simulink library "inp"  (R2021b)
settings: Solver=VariableStepAuto  StartTime=0.0  StopTime=10.0  RelTol=1e-3
undefined symbols (not defined in the file): C_TASK_5MS_S, FALSE, KINP_AcoreReadyToSlp_flg_ovrdflg, KINP_AcoreReadyToSlp_flg_ovrdval, KINP_AllowMovThd_OTA_enum_ovrdflg, KINP_AllowMovThd_OTA_enum_ovrdval, KINP_APSAngleTarget_Deg_ovrdflg, KINP_APSAngleTarget_Deg_ovrdval, KINP_APSDecReq_mps2_ovrdflg, KINP_APSDecReq_mps2_ovrdval, KINP_APSDecReqA_flg_ovrdflg, KINP_APSDecReqA_flg_ovrdval, KINP_APSDFLL_cm_ovrdflg, KINP_APSDFLL_cm_ovrdval, KINP_APSDFLR_cm_ovrdflg, KINP_APSDFLR_cm_ovrdval, KINP_APSDRLL_cm_ovrdflg, KINP_APSDRLL_cm_ovrdval, KINP_APSDRLR_cm_ovrdflg, KINP_APSDRLR_cm_ovrdval, KINP_APSExitCondition_enum_ovrdflg, KINP_APSExitCondition_enum_ovrdval, KINP_APSHWVer_enum_ovrdflg, KINP_APSHWVer_enum_ovrdval, KINP_APSProgressPCT_pct_ovrdflg, KINP_APSProgressPCT_pct_ovrdval, KINP_APSPwrReq_enum_ovrdflg, KINP_APSPwrReq_enum_ovrdval, KINP_APSReq_enum_ovrdflg, KINP_APSReq_enum_ovrdval, KINP_APSRQDisplay_enum_ovrdflg, KINP_APSRQDisplay_enum_ovrdval, KINP_APSRqEPASCtrl_flg_ovrdflg, KINP_APSRqEPASCtrl_flg_ovrdval, KINP_APSShiftPosnReq_enum_ovrdval, KINP_APSShiftPosnReq_enum_ovrflg, KINP_APSSpeedCMD_kph_ovrdval, KINP_APSSpeedCMD_kph_ovrflg, KINP_APSStaSystem_enum_ovrdflg, KINP_APSStaSystem_enum_ovrdval, KINP_APSSWVer_enum_ovrdflg, KINP_APSSWVer_enum_ovrdval, KINP_APSVMCReqA_flg_ovrdval, KINP_APSVMCReqA_flg_ovrflg, KINP_APSVRqEPASCtrl_flg_ovrdflg, KINP_APSVRqEPASCtrl_flg_ovrdval, KINP_AuxBattVolmV_mV_ovrdflg, KINP_AuxBattVolmV_mV_ovrdval, KINP_CAASSta_enum_ovrdflg, KINP_CAASSta_enum_ovrdval, KINP_CAASVMCReqA_flg_ovrdval, KINP_CAASVMCReqA_flg_ovrflg, KINP_CAN1BusOff_flg_ovrdflg, KINP_CAN1BusOff_flg_ovrdval, KINP_CAN2BusOff_flg_ovrdflg, KINP_CAN2BusOff_flg_ovrdval, KINP_CAN3BusOff_flg_ovrdflg, KINP_CAN3BusOff_flg_ovrdval, KINP_CAN4BusOff_flg_ovrdflg, KINP_CAN4BusOff_flg_ovrdval ... (+152)
libraries: FVT_lib x1037, hcu_lib x1
(part 15 of 34)

== system inp/INP/CAN1/SignalCheck/ESC5 ==
  BHAL_outputs : Inport
  inp_CanValid_bus : Inport  Port=2
  ACCAvail : FVT_lib/inp/can_signal_template  SystemSampleTime=-1  VariantActivationTime=update diagram  Latency=0  AutoFrameSizeCalculation=off
      link override defval: Value=KINP_ACCAvail_flg_defval
      link override ovrdflg: Value=KINP_ACCAvail_flg_ovrdflg
      link override ovrdval: Value=KINP_ACCAvail_flg_ovrdval
  AEBAvail : FVT_lib/inp/can_signal_template  SystemSampleTime=-1  VariantActivationTime=update diagram  Latency=0  AutoFrameSizeCalculation=off
      link override defval: Value=KINP_AEBAvail_flg_defval
      link override ovrdflg: Value=KINP_AEBAvail_flg_ovrdflg
      link override ovrdval: Value=KINP_AEBAvail_flg_ovrdval
  ActBrkLampSta : FVT_lib/inp/can_signal_template  SystemSampleTime=-1  VariantActivationTime=update diagram  Latency=0  AutoFrameSizeCalculation=off
      link override defval: Value=KINP_ActBrkLampSta_flg_defval
      link override ovrdflg: Value=KINP_ActBrkLampSta_flg_ovrdflg
      link override ovrdval: Value=KINP_ActBrkLampSta_flg_ovrdval
  BrkDiscTempSta : FVT_lib/inp/can_signal_template  SystemSampleTime=-1  VariantActivationTime=update diagram  Latency=0  AutoFrameSizeCalculation=off
      link override defval: Value=KINP_BrkDiscTempSta_flg_defval
      link override ovrdflg: Value=KINP_BrkDiscTempSta_flg_ovrdflg
      link override ovrdval: Value=KINP_BrkDiscTempSta_flg_ovrdval
  BrkPedalPos : FVT_lib/inp/can_signal_template  SystemSampleTime=-1  VariantActivationTime=update diagram  Latency=0  AutoFrameSizeCalculation=off
      link override defval: Value=KINP_BrkPedalPos_pct_defval
      link override ovrdflg: Value=KINP_BrkPedalPos_pct_ovrdflg
      link override ovrdval: Value=KINP_BrkPedalPos_pct_ovrdval
  BrkPedalPosSta : FVT_lib/inp/can_signal_template  SystemSampleTime=-1  VariantActivationTime=update diagram  Latency=0  AutoFrameSizeCalculation=off
      link override defval: Value=KINP_BrkPedalPosSta_flg_defval
      link override ovrdflg: Value=KINP_BrkPedalPosSta_flg_ovrdflg
      link override ovrdval: Value=KINP_BrkPedalPosSta_flg_ovrdval
  BrkSwSta : FVT_lib/inp/can_signal_template  SystemSampleTime=-1  VariantActivationTime=update diagram  Latency=0  AutoFrameSizeCalculation=off
      link override defval: Value=KINP_BrkSwSta_flg_defval
      link override ovrdflg: Value=KINP_BrkSwSta_flg_ovrdflg
      link override ovrdval: Value=KINP_BrkSwSta_flg_ovrdval
  BrkSwV : FVT_lib/inp/can_signal_template  SystemSampleTime=-1  VariantActivationTime=update diagram  Latency=0  AutoFrameSizeCalculation=off
      link override defval: Value=KINP_BrkSwV_flg_defval
      link override ovrdflg: Value=KINP_BrkSwV_flg_ovrdflg
      link override ovrdval: Value=KINP_BrkSwV_flg_ovrdval
  ESC5CS : FVT_lib/inp/can_signal_template  SystemSampleTime=-1  VariantActivationTime=update diagram  Latency=0  AutoFrameSizeCalculation=off
      link override defval: Value=KINP_ESC5CS_enum_defval
      link override ovrdflg: Value=KINP_ESC5CS_enum_ovrdflg
      link override ovrdval: Value=KINP_ESC5CS_enum_ovrdval
  ESC5CSErr : FVT_lib/inp/can_signal_template  SystemSampleTime=-1  VariantActivationTime=update diagram  Latency=0  AutoFrameSizeCalculation=off
      link override defval: Value=KINP_ESC5CSErr_flg_defval
      link override ovrdflg: Value=KINP_ESC5CSErr_flg_ovrdflg
      link override ovrdval: Value=KINP_ESC5CSErr_flg_ovrdval
  ESC5RC : FVT_lib/inp/can_signal_template  SystemSampleTime=-1  VariantActivationTime=update diagram  Latency=0  AutoFrameSizeCalculation=off
      link override defval: Value=KINP_ESC5RC_enum_defval
      link override ovrdflg: Value=KINP_ESC5RC_enum_ovrdflg
      link override ovrdval: Value=KINP_ESC5RC_enum_ovrdval
  ESC5RCErr : FVT_lib/inp/can_signal_template  SystemSampleTime=-1  VariantActivationTime=update diagram  Latency=0  AutoFrameSizeCalculation=off
      link override defval: Value=KINP_ESC5RCErr_flg_defval
      link override ovrdflg: Value=KINP_ESC5RCErr_flg_ovrdflg
      link override ovrdval: Value=KINP_ESC5RCErr_flg_ovrdval
  ESCADASSta : FVT_lib/inp/can_signal_template  SystemSampleTime=-1  VariantActivationTime=update diagram  Latency=0  AutoFrameSizeCalculation=off
      link override defval: Value=KINP_ESCADASSta_enum_defval
      link override ovrdflg: Value=KINP_ESCADASSta_enum_ovrdflg
      link override ovrdval: Value=KINP_ESCADASSta_enum_ovrdval
  ESCAPSSta : FVT_lib/inp/can_signal_template  SystemSampleTime=-1  VariantActivationTime=update diagram  Latency=0  AutoFrameSizeCalculation=off
      link override defval: Value=KINP_ESCAPSSta_enum_defval
      link override ovrdflg: Value=KINP_ESCAPSSta_enum_ovrdflg
      link override ovrdval: Value=KINP_ESCAPSSta_enum_ovrdval
  ESCStandstill : FVT_lib/inp/can_signal_template  SystemSampleTime=-1  VariantActivationTime=update diagram  Latency=0  AutoFrameSizeCalculation=off
      link override defval: Value=KINP_ESCStandstill_flg_defval
      link override ovrdflg: Value=KINP_ESCStandstill_flg_ovrdflg
      link override ovrdval: Value=KINP_ESCStandstill_flg_ovrdval
  FrRBCActive : FVT_lib/inp/can_signal_template  SystemSampleTime=-1  VariantActivationTime=update diagram  Latency=0  AutoFrameSizeCalculation=off
      link override defval: Value=KINP_FrRBCActive_flg_defval
      link override ovrdflg: Value=KINP_FrRBCActive_flg_ovrdflg
      link override ovrdval: Value=KINP_FrRBCActive_flg_ovrdval
  FrntAxlTrqReqBrk : FVT_lib/inp/can_signal_template  SystemSampleTime=-1  VariantActivationTime=update diagram  Latency=0  AutoFrameSizeCalculation=off
      link override defval: Value=KINP_FrntAxlTrqReqBrk_Nm_defval
      link override ovrdflg: Value=KINP_FrntAxlTrqReqBrk_Nm_ovrdflg
      link override ovrdval: Value=KINP_FrntAxlTrqReqBrk_Nm_ovrdval
  LatAccel : FVT_lib/inp/can_signal_template  SystemSampleTime=-1  VariantActivationTime=update diagram  Latency=0  AutoFrameSizeCalculation=off
      link override defval: Value=KINP_LatAccel_Gps_defval
      link override ovrdflg: Value=KINP_LatAccel_Gps_ovrdflg
      link override ovrdval: Value=KINP_LatAccel_Gps_ovrdval
  LatAccelV : FVT_lib/inp/can_signal_template  SystemSampleTime=-1  VariantActivationTime=update diagram  Latency=0  AutoFrameSizeCalculation=off
      link override defval: Value=KINP_LatAccelV_flg_defval
      link override ovrdflg: Value=KINP_LatAccelV_flg_ovrdflg
      link override ovrdval: Value=KINP_LatAccelV_flg_ovrdval
  LongAccel : FVT_lib/inp/can_signal_template  SystemSampleTime=-1  VariantActivationTime=update diagram  Latency=0  AutoFrameSizeCalculation=off
      link override defval: Value=KINP_LongAccel_Gps_defval
      link override ovrdflg: Value=KINP_LongAccel_Gps_ovrdflg
      link override ovrdval: Value=KINP_LongAccel_Gps_ovrdval
  LongAccelV : FVT_lib/inp/can_signal_template  SystemSampleTime=-1  VariantActivationTime=update diagram  Latency=0  AutoFrameSizeCalculation=off
      link override defval: Value=KINP_LongAccelV_flg_defval
      link override ovrdflg: Value=KINP_LongAccelV_flg_ovrdflg
      link override ovrdval: Value=KINP_LongAccelV_flg_ovrdval
  MCPressure : FVT_lib/inp/can_signal_template  SystemSampleTime=-1  VariantActivationTime=update diagram  Latency=0  AutoFrameSizeCalculation=off
      link override defval: Value=KINP_MCPressure_bar_defval
      link override ovrdflg: Value=KINP_MCPressure_bar_ovrdflg
      link override ovrdval: Value=KINP_MCPressure_bar_ovrdval
  MCPressureV : FVT_lib/inp/can_signal_template  SystemSampleTime=-1  VariantActivationTime=update diagram  Latency=0  AutoFrameSizeCalculation=off
      link override defval: Value=KINP_MCPressureV_flg_defval
      link override ovrdflg: Value=KINP_MCPressureV_flg_ovrdflg
      link override ovrdval: Value=KINP_MCPressureV_flg_ovrdval
  MeterIndVehSpeed : FVT_lib/inp/can_signal_template  SystemSampleTime=-1  VariantActivationTime=update diagram  Latency=0  AutoFrameSizeCalculation=off
      link override defval: Value=KINP_MeterIndVehSpeed_kph_defval
      link override ovrdflg: Value=KINP_MeterIndVehSpeed_kph_ovrdflg
      link override ovrdval: Value=KINP_MeterIndVehSpeed_kph_ovrdval
  RDCActive : FVT_lib/inp/can_signal_template  SystemSampleTime=-1  VariantActivationTime=update diagram  Latency=0  AutoFrameSizeCalculation=off
      link override defval: Value=KINP_RDCActive_enum_defval
      link override ovrdflg: Value=KINP_RDCActive_enum_ovrdflg
      link override ovrdval: Value=KINP_RDCActive_enum_ovrdval
  RearAxlTrqReqBrk : FVT_lib/inp/can_signal_template  SystemSampleTime=-1  VariantActivationTime=update diagram  Latency=0  AutoFrameSizeCalculation=off
      link override defval: Value=KINP_RearAxlTrqReqBrk_Nm_defval
      link override ovrdflg: Value=KINP_RearAxlTrqReqBrk_Nm_ovrdflg
      link override ovrdval: Value=KINP_RearAxlTrqReqBrk_Nm_ovrdval
  RrRBCActive : FVT_lib/inp/can_signal_template  SystemSampleTime=-1  VariantActivationTime=update diagram  Latency=0  AutoFrameSizeCalculation=off
      link override defval: Value=KINP_RrRBCActive_flg_defval
      link override ovrdflg: Value=KINP_RrRBCActive_flg_ovrdflg
      link override ovrdval: Value=KINP_RrRBCActive_flg_ovrdval
  Terminator_{1..29} (29 alike) : Terminator
  True_VHAL_ACCAvail_flg : Constant  Value=TRUE  OutDataTypeStr=boolean
  True_VHAL_AEBAvail_flg : Constant  Value=TRUE  OutDataTypeStr=boolean
  True_VHAL_ActBrkLampSta_flg : Constant  Value=TRUE  OutDataTypeStr=boolean
  True_VHAL_BrkDiscTempSta_flg : Constant  Value=TRUE  OutDataTypeStr=boolean
  True_VHAL_BrkPedalPosSta_flg : Constant  Value=TRUE  OutDataTypeStr=boolean
  True_VHAL_BrkPedalPos_pct : Constant  Value=TRUE  OutDataTypeStr=boolean
  True_VHAL_BrkSwSta_flg : Constant  Value=TRUE  OutDataTypeStr=boolean
  True_VHAL_BrkSwV_flg : Constant  Value=TRUE  OutDataTypeStr=boolean
  True_VHAL_ESC5CSErr_flg : Constant  Value=TRUE  OutDataTypeStr=boolean
  True_VHAL_ESC5CS_enum : Constant  Value=TRUE  OutDataTypeStr=boolean
  True_VHAL_ESC5RCErr_flg : Constant  Value=TRUE  OutDataTypeStr=boolean
  True_VHAL_ESC5RC_enum : Constant  Value=TRUE  OutDataTypeStr=boolean
  True_VHAL_ESCADASSta_enum : Constant  Value=TRUE  OutDataTypeStr=boolean
  True_VHAL_ESCAPSSta_enum : Constant  Value=TRUE  OutDataTypeStr=boolean
  True_VHAL_ESCStandstill_flg : Constant  Value=TRUE  OutDataTypeStr=boolean
  True_VHAL_FrRBCActive_flg : Constant  Value=TRUE  OutDataTypeStr=boolean
  True_VHAL_FrntAxlTrqReqBrk_Nm : Constant  Value=TRUE  OutDataTypeStr=boolean
  True_VHAL_LatAccelV_flg : Constant  Value=TRUE  OutDataTypeStr=boolean
  True_VHAL_LatAccel_Gps : Constant  Value=TRUE  OutDataTypeStr=boolean
  True_VHAL_LongAccelV_flg : Constant  Value=TRUE  OutDataTypeStr=boolean
  True_VHAL_LongAccel_Gps : Constant  Value=TRUE  OutDataTypeStr=boolean
  True_VHAL_MCPressureV_flg : Constant  Value=TRUE  OutDataTypeStr=boolean
  True_VHAL_MCPressure_bar : Constant  Value=TRUE  OutDataTypeStr=boolean
  True_VHAL_MeterIndVehSpeed_kph : Constant  Value=TRUE  OutDataTypeStr=boolean
  True_VHAL_RDCActive_enum : Constant  Value=TRUE  OutDataTypeStr=boolean
  True_VHAL_RearAxlTrqReqBrk_Nm : Constant  Value=TRUE  OutDataTypeStr=boolean
  True_VHAL_RrRBCActive_flg : Constant  Value=TRUE  OutDataTypeStr=boolean
  True_VHAL_YawRateV_flg : Constant  Value=TRUE  OutDataTypeStr=boolean
  True_VHAL_YawRate_degps : Constant  Value=TRUE  OutDataTypeStr=boolean
  YawRate : FVT_lib/inp/can_signal_template  SystemSampleTime=-1  VariantActivationTime=update diagram  Latency=0  AutoFrameSizeCalculation=off
      link override defval: Value=KINP_YawRate_degps_defval
      link override ovrdflg: Value=KINP_YawRate_degps_ovrdflg
      link override ovrdval: Value=KINP_YawRate_degps_ovrdval
  YawRateV : FVT_lib/inp/can_signal_template  SystemSampleTime=-1  VariantActivationTime=update diagram  Latency=0  AutoFrameSizeCalculation=off
      link override defval: Value=KINP_YawRateV_flg_defval
      link override ovrdflg: Value=KINP_YawRateV_flg_ovrdflg
      link override ovrdval: Value=KINP_YawRateV_flg_ovrdval
  slr1_{1..29} (29 alike) : BusSelector  OutputSignals=VINP_CANMsgValidESC5_flg
  slr_VHAL_ACCAvail_flg : BusSelector  OutputSignals=VHAL_ACCAvail_flg
  slr_VHAL_AEBAvail_flg : BusSelector  OutputSignals=VHAL_AEBAvail_flg
  slr_VHAL_ActBrkLampSta_flg : BusSelector  OutputSignals=VHAL_ActBrkLampSta_flg
  slr_VHAL_BrkDiscTempSta_flg : BusSelector  OutputSignals=VHAL_BrkDiscTempSta_flg
  slr_VHAL_BrkPedalPosSta_flg : BusSelector  OutputSignals=VHAL_BrkPedalPosSta_flg
  slr_VHAL_BrkPedalPos_pct : BusSelector  OutputSignals=VHAL_BrkPedalPos_pct
  slr_VHAL_BrkSwSta_flg : BusSelector  OutputSignals=VHAL_BrkSwSta_flg
  slr_VHAL_BrkSwV_flg : BusSelector  OutputSignals=VHAL_BrkSwV_flg
  slr_VHAL_ESC5CSErr_flg : BusSelector  OutputSignals=VHAL_ESC5CSErr_flg
  slr_VHAL_ESC5CS_enum : BusSelector  OutputSignals=VHAL_ESC5CS_enum
  slr_VHAL_ESC5RCErr_flg : BusSelector  OutputSignals=VHAL_ESC5RCErr_flg
  slr_VHAL_ESC5RC_enum : BusSelector  OutputSignals=VHAL_ESC5RC_enum
  slr_VHAL_ESCADASSta_enum : BusSelector  OutputSignals=VHAL_ESCADASSta_enum
  slr_VHAL_ESCAPSSta_enum : BusSelector  OutputSignals=VHAL_ESCAPSSta_enum
  slr_VHAL_ESCStandstill_flg : BusSelector  OutputSignals=VHAL_ESCStandstill_flg
  slr_VHAL_FrRBCActive_flg : BusSelector  OutputSignals=VHAL_FrRBCActive_flg
  slr_VHAL_FrntAxlTrqReqBrk_Nm : BusSelector  OutputSignals=VHAL_FrntAxlTrqReqBrk_Nm
  slr_VHAL_LatAccelV_flg : BusSelector  OutputSignals=VHAL_LatAccelV_flg
  slr_VHAL_LatAccel_Gps : BusSelector  OutputSignals=VHAL_LatAccel_Gps
  slr_VHAL_LongAccelV_flg : BusSelector  OutputSignals=VHAL_LongAccelV_flg
  slr_VHAL_LongAccel_Gps : BusSelector  OutputSignals=VHAL_LongAccel_Gps
  slr_VHAL_MCPressureV_flg : BusSelector  OutputSignals=VHAL_MCPressureV_flg
  slr_VHAL_MCPressure_bar : BusSelector  OutputSignals=VHAL_MCPressure_bar
  slr_VHAL_MeterIndVehSpeed_kph : BusSelector  OutputSignals=VHAL_MeterIndVehSpeed_kph
  slr_VHAL_RDCActive_enum : BusSelector  OutputSignals=VHAL_RDCActive_enum
  slr_VHAL_RearAxlTrqReqBrk_Nm : BusSelector  OutputSignals=VHAL_RearAxlTrqReqBrk_Nm
  slr_VHAL_RrRBCActive_flg : BusSelector  OutputSignals=VHAL_RrRBCActive_flg
  slr_VHAL_YawRateV_flg : BusSelector  OutputSignals=VHAL_YawRateV_flg
  slr_VHAL_YawRate_degps : BusSelector  OutputSignals=VHAL_YawRate_degps
  VINP_ESC5CSErr_flg : Outport
  VINP_ESC5RCErr_flg : Outport  Port=2
  VINP_ACCAvail_flg : Outport  Port=3
  VINP_AEBAvail_flg : Outport  Port=4
  VINP_ActBrkLampSta_flg : Outport  Port=5
  VINP_BrkDiscTempSta_flg : Outport  Port=6
  VINP_BrkPedalPos_pct : Outport  Port=7
  VINP_BrkPedalPosSta_flg : Outport  Port=8
  VINP_BrkSwSta_flg : Outport  Port=9
  VINP_BrkSwV_flg : Outport  Port=10
  VINP_ESC5CS_enum : Outport  Port=11
  VINP_ESC5RC_enum : Outport  Port=12
  VINP_ESCADASSta_enum : Outport  Port=13
  VINP_ESCAPSSta_enum : Outport  Port=14
  VINP_ESCStandstill_flg : Outport  Port=15
  VINP_FrRBCActive_flg : Outport  Port=16
  VINP_FrntAxlTrqReqBrk_Nm : Outport  Port=17
  VINP_LatAccel_Gps : Outport  Port=18
  VINP_LatAccelV_flg : Outport  Port=19
  VINP_LongAccel_Gps : Outport  Port=20
  VINP_LongAccelV_flg : Outport  Port=21
  VINP_MCPressure_bar : Outport  Port=22
  VINP_MCPressureV_flg : Outport  Port=23
  VINP_MeterIndVehSpeed_kph : Outport  Port=24
  VINP_RDCActive_enum : Outport  Port=25
  VINP_RearAxlTrqReqBrk_Nm : Outport  Port=26
  VINP_RrRBCActive_flg : Outport  Port=27
  VINP_YawRate_degps : Outport  Port=28
  VINP_YawRateV_flg : Outport  Port=29
  wires:
  BHAL_outputs/1 -> [BHAL_outputs]
  inp_CanValid_bus/1 -> [inp_CanValid_bus]
  [BHAL_outputs] -> slr_VHAL_ESC5CSErr_flg/1
  slr_VHAL_ESC5CSErr_flg/1 -> ESC5CSErr/1  "<VHAL_ESC5CSErr_flg>"
  True_VHAL_ESC5CSErr_flg/1 -> ESC5CSErr/2
  [inp_CanValid_bus] -> slr1_1/1
  slr1_1/1 -> ESC5CSErr/3  "<VINP_CANMsgValidESC5_flg>"
  ESC5CSErr/1 -> VINP_ESC5CSErr_flg/1  "VINP_ESC5CSErr_flg"
  ESC5CSErr/2 -> Terminator_1/1
  [BHAL_outputs] -> slr_VHAL_ESC5RCErr_flg/1
  slr_VHAL_ESC5RCErr_flg/1 -> ESC5RCErr/1  "<VHAL_ESC5RCErr_flg>"
  True_VHAL_ESC5RCErr_flg/1 -> ESC5RCErr/2
  [inp_CanValid_bus] -> slr1_2/1
  slr1_2/1 -> ESC5RCErr/3  "<VINP_CANMsgValidESC5_flg>"
  ESC5RCErr/1 -> VINP_ESC5RCErr_flg/1  "VINP_ESC5RCErr_flg"
  ESC5RCErr/2 -> Terminator_2/1
  [BHAL_outputs] -> slr_VHAL_ACCAvail_flg/1
  slr_VHAL_ACCAvail_flg/1 -> ACCAvail/1  "<VHAL_ACCAvail_flg>"
  True_VHAL_ACCAvail_flg/1 -> ACCAvail/2
  [inp_CanValid_bus] -> slr1_3/1
  slr1_3/1 -> ACCAvail/3  "<VINP_CANMsgValidESC5_flg>"
  ACCAvail/1 -> VINP_ACCAvail_flg/1  "VINP_ACCAvail_flg"
  ACCAvail/2 -> Terminator_3/1
  [BHAL_outputs] -> slr_VHAL_AEBAvail_flg/1
  slr_VHAL_AEBAvail_flg/1 -> AEBAvail/1  "<VHAL_AEBAvail_flg>"
  True_VHAL_AEBAvail_flg/1 -> AEBAvail/2
  [inp_CanValid_bus] -> slr1_4/1
  slr1_4/1 -> AEBAvail/3  "<VINP_CANMsgValidESC5_flg>"
  AEBAvail/1 -> VINP_AEBAvail_flg/1  "VINP_AEBAvail_flg"
  AEBAvail/2 -> Terminator_4/1
  [BHAL_outputs] -> slr_VHAL_ActBrkLampSta_flg/1
  slr_VHAL_ActBrkLampSta_flg/1 -> ActBrkLampSta/1  "<VHAL_ActBrkLampSta_flg>"
  True_VHAL_ActBrkLampSta_flg/1 -> ActBrkLampSta/2
  [inp_CanValid_bus] -> slr1_5/1
  slr1_5/1 -> ActBrkLampSta/3  "<VINP_CANMsgValidESC5_flg>"
  ActBrkLampSta/1 -> VINP_ActBrkLampSta_flg/1  "VINP_ActBrkLampSta_flg"
  ActBrkLampSta/2 -> Terminator_5/1
  [BHAL_outputs] -> slr_VHAL_BrkDiscTempSta_flg/1
  slr_VHAL_BrkDiscTempSta_flg/1 -> BrkDiscTempSta/1  "<VHAL_BrkDiscTempSta_flg>"
  True_VHAL_BrkDiscTempSta_flg/1 -> BrkDiscTempSta/2
  [inp_CanValid_bus] -> slr1_6/1
  slr1_6/1 -> BrkDiscTempSta/3  "<VINP_CANMsgValidESC5_flg>"
  BrkDiscTempSta/1 -> VINP_BrkDiscTempSta_flg/1  "VINP_BrkDiscTempSta_flg"
  BrkDiscTempSta/2 -> Terminator_6/1
  [BHAL_outputs] -> slr_VHAL_BrkPedalPos_pct/1
  slr_VHAL_BrkPedalPos_pct/1 -> BrkPedalPos/1  "<VHAL_BrkPedalPos_pct>"
  True_VHAL_BrkPedalPos_pct/1 -> BrkPedalPos/2
  [inp_CanValid_bus] -> slr1_7/1
  slr1_7/1 -> BrkPedalPos/3  "<VINP_CANMsgValidESC5_flg>"
  BrkPedalPos/1 -> VINP_BrkPedalPos_pct/1  "VINP_BrkPedalPos_pct"
  BrkPedalPos/2 -> Terminator_7/1
  [BHAL_outputs] -> slr_VHAL_BrkPedalPosSta_flg/1
  slr_VHAL_BrkPedalPosSta_flg/1 -> BrkPedalPosSta/1  "<VHAL_BrkPedalPosSta_flg>"
  True_VHAL_BrkPedalPosSta_flg/1 -> BrkPedalPosSta/2
  [inp_CanValid_bus] -> slr1_8/1
  slr1_8/1 -> BrkPedalPosSta/3  "<VINP_CANMsgValidESC5_flg>"
  BrkPedalPosSta/1 -> VINP_BrkPedalPosSta_flg/1  "VINP_BrkPedalPosSta_flg"
  BrkPedalPosSta/2 -> Terminator_8/1
  [BHAL_outputs] -> slr_VHAL_BrkSwSta_flg/1
  slr_VHAL_BrkSwSta_flg/1 -> BrkSwSta/1  "<VHAL_BrkSwSta_flg>"
  True_VHAL_BrkSwSta_flg/1 -> BrkSwSta/2
  [inp_CanValid_bus] -> slr1_9/1
  slr1_9/1 -> BrkSwSta/3  "<VINP_CANMsgValidESC5_flg>"
  BrkSwSta/1 -> VINP_BrkSwSta_flg/1  "VINP_BrkSwSta_flg"
  BrkSwSta/2 -> Terminator_9/1
  [BHAL_outputs] -> slr_VHAL_BrkSwV_flg/1
  slr_VHAL_BrkSwV_flg/1 -> BrkSwV/1  "<VHAL_BrkSwV_flg>"
  True_VHAL_BrkSwV_flg/1 -> BrkSwV/2
  [inp_CanValid_bus] -> slr1_10/1
  slr1_10/1 -> BrkSwV/3  "<VINP_CANMsgValidESC5_flg>"
  BrkSwV/1 -> VINP_BrkSwV_flg/1  "VINP_BrkSwV_flg"
  BrkSwV/2 -> Terminator_10/1
  [BHAL_outputs] -> slr_VHAL_ESC5CS_enum/1
  slr_VHAL_ESC5CS_enum/1 -> ESC5CS/1  "<VHAL_ESC5CS_enum>"
  True_VHAL_ESC5CS_enum/1 -> ESC5CS/2
  [inp_CanValid_bus] -> slr1_11/1
  slr1_11/1 -> ESC5CS/3  "<VINP_CANMsgValidESC5_flg>"
  ESC5CS/1 -> VINP_ESC5CS_enum/1  "VINP_ESC5CS_enum"
  ESC5CS/2 -> Terminator_11/1
  [BHAL_outputs] -> slr_VHAL_ESC5RC_enum/1
  slr_VHAL_ESC5RC_enum/1 -> ESC5RC/1  "<VHAL_ESC5RC_enum>"
  True_VHAL_ESC5RC_enum/1 -> ESC5RC/2
  [inp_CanValid_bus] -> slr1_12/1
  slr1_12/1 -> ESC5RC/3  "<VINP_CANMsgValidESC5_flg>"
  ESC5RC/1 -> VINP_ESC5RC_enum/1  "VINP_ESC5RC_enum"
  ESC5RC/2 -> Terminator_12/1
  [BHAL_outputs] -> slr_VHAL_ESCADASSta_enum/1
  slr_VHAL_ESCADASSta_enum/1 -> ESCADASSta/1  "<VHAL_ESCADASSta_enum>"
  True_VHAL_ESCADASSta_enum/1 -> ESCADASSta/2
  [inp_CanValid_bus] -> slr1_13/1
  slr1_13/1 -> ESCADASSta/3  "<VINP_CANMsgValidESC5_flg>"
  ESCADASSta/1 -> VINP_ESCADASSta_enum/1  "VINP_ESCADASSta_enum"
  ESCADASSta/2 -> Terminator_13/1
  [BHAL_outputs] -> slr_VHAL_ESCAPSSta_enum/1
  slr_VHAL_ESCAPSSta_enum/1 -> ESCAPSSta/1  "<VHAL_ESCAPSSta_enum>"
  True_VHAL_ESCAPSSta_enum/1 -> ESCAPSSta/2
  [inp_CanValid_bus] -> slr1_14/1
  slr1_14/1 -> ESCAPSSta/3  "<VINP_CANMsgValidESC5_flg>"
  ESCAPSSta/1 -> VINP_ESCAPSSta_enum/1  "VINP_ESCAPSSta_enum"
  ESCAPSSta/2 -> Terminator_14/1
  [BHAL_outputs] -> slr_VHAL_ESCStandstill_flg/1
  slr_VHAL_ESCStandstill_flg/1 -> ESCStandstill/1  "<VHAL_ESCStandstill_flg>"
  True_VHAL_ESCStandstill_flg/1 -> ESCStandstill/2
  [inp_CanValid_bus] -> slr1_15/1
  slr1_15/1 -> ESCStandstill/3  "<VINP_CANMsgValidESC5_flg>"
  ESCStandstill/1 -> VINP_ESCStandstill_flg/1  "VINP_ESCStandstill_flg"
  ESCStandstill/2 -> Terminator_15/1
  [BHAL_outputs] -> slr_VHAL_FrRBCActive_flg/1
  slr_VHAL_FrRBCActive_flg/1 -> FrRBCActive/1  "<VHAL_FrRBCActive_flg>"
  True_VHAL_FrRBCActive_flg/1 -> FrRBCActive/2
  [inp_CanValid_bus] -> slr1_16/1
  slr1_16/1 -> FrRBCActive/3  "<VINP_CANMsgValidESC5_flg>"
  FrRBCActive/1 -> VINP_FrRBCActive_flg/1  "VINP_FrRBCActive_flg"
  FrRBCActive/2 -> Terminator_16/1
  [BHAL_outputs] -> slr_VHAL_FrntAxlTrqReqBrk_Nm/1
  slr_VHAL_FrntAxlTrqReqBrk_Nm/1 -> FrntAxlTrqReqBrk/1  "<VHAL_FrntAxlTrqReqBrk_Nm>"
  True_VHAL_FrntAxlTrqReqBrk_Nm/1 -> FrntAxlTrqReqBrk/2
  [inp_CanValid_bus] -> slr1_17/1
  slr1_17/1 -> FrntAxlTrqReqBrk/3  "<VINP_CANMsgValidESC5_flg>"
  FrntAxlTrqReqBrk/1 -> VINP_FrntAxlTrqReqBrk_Nm/1  "VINP_FrntAxlTrqReqBrk_Nm"
  FrntAxlTrqReqBrk/2 -> Terminator_17/1
  [BHAL_outputs] -> slr_VHAL_LatAccel_Gps/1
  slr_VHAL_LatAccel_Gps/1 -> LatAccel/1  "<VHAL_LatAccel_Gps>"
  True_VHAL_LatAccel_Gps/1 -> LatAccel/2
  [inp_CanValid_bus] -> slr1_18/1
  slr1_18/1 -> LatAccel/3  "<VINP_CANMsgValidESC5_flg>"
  LatAccel/1 -> VINP_LatAccel_Gps/1  "VINP_LatAccel_Gps"
  LatAccel/2 -> Terminator_18/1
  [BHAL_outputs] -> slr_VHAL_LatAccelV_flg/1
  slr_VHAL_LatAccelV_flg/1 -> LatAccelV/1  "<VHAL_LatAccelV_flg>"
  True_VHAL_LatAccelV_flg/1 -> LatAccelV/2
  [inp_CanValid_bus] -> slr1_19/1
  slr1_19/1 -> LatAccelV/3  "<VINP_CANMsgValidESC5_flg>"
  LatAccelV/1 -> VINP_LatAccelV_flg/1  "VINP_LatAccelV_flg"
  LatAccelV/2 -> Terminator_19/1
  [BHAL_outputs] -> slr_VHAL_LongAccel_Gps/1
  slr_VHAL_LongAccel_Gps/1 -> LongAccel/1  "<VHAL_LongAccel_Gps>"
  True_VHAL_LongAccel_Gps/1 -> LongAccel/2
  [inp_CanValid_bus] -> slr1_20/1
  slr1_20/1 -> LongAccel/3  "<VINP_CANMsgValidESC5_flg>"
  LongAccel/1 -> VINP_LongAccel_Gps/1  "VINP_LongAccel_Gps"
  LongAccel/2 -> Terminator_20/1
  [BHAL_outputs] -> slr_VHAL_LongAccelV_flg/1
  slr_VHAL_LongAccelV_flg/1 -> LongAccelV/1  "<VHAL_LongAccelV_flg>"
  True_VHAL_LongAccelV_flg/1 -> LongAccelV/2
  [inp_CanValid_bus] -> slr1_21/1
  slr1_21/1 -> LongAccelV/3  "<VINP_CANMsgValidESC5_flg>"
  LongAccelV/1 -> VINP_LongAccelV_flg/1  "VINP_LongAccelV_flg"
  LongAccelV/2 -> Terminator_21/1
  [BHAL_outputs] -> slr_VHAL_MCPressure_bar/1
  slr_VHAL_MCPressure_bar/1 -> MCPressure/1  "<VHAL_MCPressure_bar>"
  True_VHAL_MCPressure_bar/1 -> MCPressure/2
  [inp_CanValid_bus] -> slr1_22/1
  slr1_22/1 -> MCPressure/3  "<VINP_CANMsgValidESC5_flg>"
  MCPressure/1 -> VINP_MCPressure_bar/1  "VINP_MCPressure_bar"
  MCPressure/2 -> Terminator_22/1
  [BHAL_outputs] -> slr_VHAL_MCPressureV_flg/1
  slr_VHAL_MCPressureV_flg/1 -> MCPressureV/1  "<VHAL_MCPressureV_flg>"
  True_VHAL_MCPressureV_flg/1 -> MCPressureV/2
  [inp_CanValid_bus] -> slr1_23/1
  slr1_23/1 -> MCPressureV/3  "<VINP_CANMsgValidESC5_flg>"
  MCPressureV/1 -> VINP_MCPressureV_flg/1  "VINP_MCPressureV_flg"
  MCPressureV/2 -> Terminator_23/1
  [BHAL_outputs] -> slr_VHAL_MeterIndVehSpeed_kph/1
  slr_VHAL_MeterIndVehSpeed_kph/1 -> MeterIndVehSpeed/1  "<VHAL_MeterIndVehSpeed_kph>"
  True_VHAL_MeterIndVehSpeed_kph/1 -> MeterIndVehSpeed/2
  [inp_CanValid_bus] -> slr1_24/1
  slr1_24/1 -> MeterIndVehSpeed/3  "<VINP_CANMsgValidESC5_flg>"
  MeterIndVehSpeed/1 -> VINP_MeterIndVehSpeed_kph/1  "VINP_MeterIndVehSpeed_kph"
  MeterIndVehSpeed/2 -> Terminator_24/1
  [BHAL_outputs] -> slr_VHAL_RDCActive_enum/1
  slr_VHAL_RDCActive_enum/1 -> RDCActive/1  "<VHAL_RDCActive_enum>"
  True_VHAL_RDCActive_enum/1 -> RDCActive/2
  [inp_CanValid_bus] -> slr1_25/1
  slr1_25/1 -> RDCActive/3  "<VINP_CANMsgValidESC5_flg>"
  RDCActive/1 -> VINP_RDCActive_enum/1  "VINP_RDCActive_enum"
  RDCActive/2 -> Terminator_25/1
  [BHAL_outputs] -> slr_VHAL_RearAxlTrqReqBrk_Nm/1
  slr_VHAL_RearAxlTrqReqBrk_Nm/1 -> RearAxlTrqReqBrk/1  "<VHAL_RearAxlTrqReqBrk_Nm>"
  True_VHAL_RearAxlTrqReqBrk_Nm/1 -> RearAxlTrqReqBrk/2
  [inp_CanValid_bus] -> slr1_26/1
  slr1_26/1 -> RearAxlTrqReqBrk/3  "<VINP_CANMsgValidESC5_flg>"
  RearAxlTrqReqBrk/1 -> VINP_RearAxlTrqReqBrk_Nm/1  "VINP_RearAxlTrqReqBrk_Nm"
  RearAxlTrqReqBrk/2 -> Terminator_26/1
  [BHAL_outputs] -> slr_VHAL_RrRBCActive_flg/1
  slr_VHAL_RrRBCActive_flg/1 -> RrRBCActive/1  "<VHAL_RrRBCActive_flg>"
  True_VHAL_RrRBCActive_flg/1 -> RrRBCActive/2
  [inp_CanValid_bus] -> slr1_27/1
  slr1_27/1 -> RrRBCActive/3  "<VINP_CANMsgValidESC5_flg>"
  RrRBCActive/1 -> VINP_RrRBCActive_flg/1  "VINP_RrRBCActive_flg"
  RrRBCActive/2 -> Terminator_27/1
  [BHAL_outputs] -> slr_VHAL_YawRate_degps/1
  slr_VHAL_YawRate_degps/1 -> YawRate/1  "<VHAL_YawRate_degps>"
  True_VHAL_YawRate_degps/1 -> YawRate/2
  [inp_CanValid_bus] -> slr1_28/1
  slr1_28/1 -> YawRate/3  "<VINP_CANMsgValidESC5_flg>"
  YawRate/1 -> VINP_YawRate_degps/1  "VINP_YawRate_degps"
  YawRate/2 -> Terminator_28/1
  [BHAL_outputs] -> slr_VHAL_YawRateV_flg/1
  slr_VHAL_YawRateV_flg/1 -> YawRateV/1  "<VHAL_YawRateV_flg>"
  True_VHAL_YawRateV_flg/1 -> YawRateV/2
  [inp_CanValid_bus] -> slr1_29/1
  slr1_29/1 -> YawRateV/3  "<VINP_CANMsgValidESC5_flg>"
  YawRateV/1 -> VINP_YawRateV_flg/1  "VINP_YawRateV_flg"
  YawRateV/2 -> Terminator_29/1

== system inp/INP/CAN1/SignalCheck/eBST1 ==
  BHAL_outputs : Inport
  inp_CanValid_bus : Inport  Port=2
  LowBrakeFluidSta : FVT_lib/inp/can_signal_template  SystemSampleTime=-1  VariantActivationTime=update diagram  Latency=0  AutoFrameSizeCalculation=off
      link override defval: Value=KINP_LowBrakeFluidSta_flg_defval
      link override ovrdflg: Value=KINP_LowBrakeFluidSta_flg_ovrdflg
      link override ovrdval: Value=KINP_LowBrakeFluidSta_flg_ovrdval
  Terminator_{1..4} (4 alike) : Terminator
  True_VHAL_LowBrakeFluidSta_flg : Constant  Value=TRUE  OutDataTypeStr=boolean
  True_VHAL_eBSTAmberWnlmpSta_flg : Constant  Value=TRUE  OutDataTypeStr=boolean
  True_VHAL_eBSTBeepReq_flg : Constant  Value=TRUE  OutDataTypeStr=boolean
  True_VHAL_eBSTRedWnlmpSta_flg : Constant  Value=TRUE  OutDataTypeStr=boolean
  eBSTAmberWnlmpSta : FVT_lib/inp/can_signal_template  SystemSampleTime=-1  VariantActivationTime=update diagram  Latency=0  AutoFrameSizeCalculation=off
      link override defval: Value=KINP_eBSTAmberWnlmpSta_flg_defval
      link override ovrdflg: Value=KINP_eBSTAmberWnlmpSta_flg_ovrdflg
      link override ovrdval: Value=KINP_eBSTAmberWnlmpSta_flg_ovrdval
  eBSTBeepReq : FVT_lib/inp/can_signal_template  SystemSampleTime=-1  VariantActivationTime=update diagram  Latency=0  AutoFrameSizeCalculation=off
      link override defval: Value=KINP_eBSTBeepReq_flg_defval
      link override ovrdflg: Value=KINP_eBSTBeepReq_flg_ovrdflg
      link override ovrdval: Value=KINP_eBSTBeepReq_flg_ovrdval
  eBSTRedWnlmpSta : FVT_lib/inp/can_signal_template  SystemSampleTime=-1  VariantActivationTime=update diagram  Latency=0  AutoFrameSizeCalculation=off
      link override defval: Value=KINP_eBSTRedWnlmpSta_flg_defval
      link override ovrdflg: Value=KINP_eBSTRedWnlmpSta_flg_ovrdflg
      link override ovrdval: Value=KINP_eBSTRedWnlmpSta_flg_ovrdval
  slr1_{1..4} (4 alike) : BusSelector  OutputSignals=VINP_CANMsgValideBST1_flg
  slr_VHAL_LowBrakeFluidSta_flg : BusSelector  OutputSignals=VHAL_LowBrakeFluidSta_flg
  slr_VHAL_eBSTAmberWnlmpSta_flg : BusSelector  OutputSignals=VHAL_eBSTAmberWnlmpSta_flg
  slr_VHAL_eBSTBeepReq_flg : BusSelector  OutputSignals=VHAL_eBSTBeepReq_flg
  slr_VHAL_eBSTRedWnlmpSta_flg : BusSelector  OutputSignals=VHAL_eBSTRedWnlmpSta_flg
  VINP_LowBrakeFluidSta_flg : Outport
  VINP_eBSTAmberWnlmpSta_flg : Outport  Port=2
  VINP_eBSTBeepReq_flg : Outport  Port=3
  VINP_eBSTRedWnlmpSta_flg : Outport  Port=4
  wires:
  BHAL_outputs/1 -> [BHAL_outputs]
  inp_CanValid_bus/1 -> [inp_CanValid_bus]
  [BHAL_outputs] -> slr_VHAL_LowBrakeFluidSta_flg/1
  slr_VHAL_LowBrakeFluidSta_flg/1 -> LowBrakeFluidSta/1  "<VHAL_LowBrakeFluidSta_flg>"
  True_VHAL_LowBrakeFluidSta_flg/1 -> LowBrakeFluidSta/2
  [inp_CanValid_bus] -> slr1_1/1
  slr1_1/1 -> LowBrakeFluidSta/3  "<VINP_CANMsgValideBST1_flg>"
  LowBrakeFluidSta/1 -> VINP_LowBrakeFluidSta_flg/1  "VINP_LowBrakeFluidSta_flg"
  LowBrakeFluidSta/2 -> Terminator_1/1
  [BHAL_outputs] -> slr_VHAL_eBSTAmberWnlmpSta_flg/1
  slr_VHAL_eBSTAmberWnlmpSta_flg/1 -> eBSTAmberWnlmpSta/1  "<VHAL_eBSTAmberWnlmpSta_flg>"
  True_VHAL_eBSTAmberWnlmpSta_flg/1 -> eBSTAmberWnlmpSta/2
  [inp_CanValid_bus] -> slr1_2/1
  slr1_2/1 -> eBSTAmberWnlmpSta/3  "<VINP_CANMsgValideBST1_flg>"
  eBSTAmberWnlmpSta/1 -> VINP_eBSTAmberWnlmpSta_flg/1  "VINP_eBSTAmberWnlmpSta_flg"
  eBSTAmberWnlmpSta/2 -> Terminator_2/1
  [BHAL_outputs] -> slr_VHAL_eBSTBeepReq_flg/1
  slr_VHAL_eBSTBeepReq_flg/1 -> eBSTBeepReq/1  "<VHAL_eBSTBeepReq_flg>"
  True_VHAL_eBSTBeepReq_flg/1 -> eBSTBeepReq/2
  [inp_CanValid_bus] -> slr1_3/1
  slr1_3/1 -> eBSTBeepReq/3  "<VINP_CANMsgValideBST1_flg>"
  eBSTBeepReq/1 -> VINP_eBSTBeepReq_flg/1  "VINP_eBSTBeepReq_flg"
  eBSTBeepReq/2 -> Terminator_3/1
  [BHAL_outputs] -> slr_VHAL_eBSTRedWnlmpSta_flg/1
  slr_VHAL_eBSTRedWnlmpSta_flg/1 -> eBSTRedWnlmpSta/1  "<VHAL_eBSTRedWnlmpSta_flg>"
  True_VHAL_eBSTRedWnlmpSta_flg/1 -> eBSTRedWnlmpSta/2
  [inp_CanValid_bus] -> slr1_4/1
  slr1_4/1 -> eBSTRedWnlmpSta/3  "<VINP_CANMsgValideBST1_flg>"
  eBSTRedWnlmpSta/1 -> VINP_eBSTRedWnlmpSta_flg/1  "VINP_eBSTRedWnlmpSta_flg"
  eBSTRedWnlmpSta/2 -> Terminator_4/1

== system inp/INP/CAN2/SignalCheck/HMI1 ==
  BHAL_outputs : Inport
  inp_CanValid_bus : Inport  Port=2
  HMIACAirIntMCmd : FVT_lib/inp/can_signal_template  SystemSampleTime=-1  VariantActivationTime=update diagram  Latency=0  AutoFrameSizeCalculation=off
      link override defval: Value=KINP_HMIACAirIntMCmd_flg_defval
      link override ovrdflg: Value=KINP_HMIACAirIntMCmd_flg_ovrdflg
      link override ovrdval: Value=KINP_HMIACAirIntMCmd_flg_ovrdval
  HMIACAirIntPCmd : FVT_lib/inp/can_signal_template  SystemSampleTime=-1  VariantActivationTime=update diagram  Latency=0  AutoFrameSizeCalculation=off
      link override defval: Value=KINP_HMIACAirIntPCmd_flg_defval
      link override ovrdflg: Value=KINP_HMIACAirIntPCmd_flg_ovrdflg
      link override ovrdval: Value=KINP_HMIACAirIntPCmd_flg_ovrdval
  HMIACAutoBtnCmd : FVT_lib/inp/can_signal_template  SystemSampleTime=-1  VariantActivationTime=update diagram  Latency=0  AutoFrameSizeCalculation=off
      link override defval: Value=KINP_HMIACAutoBtnCmd_flg_defval
      link override ovrdflg: Value=KINP_HMIACAutoBtnCmd_flg_ovrdflg
      link override ovrdval: Value=KINP_HMIACAutoBtnCmd_flg_ovrdval
  HMIACBtnCmd : FVT_lib/inp/can_signal_template  SystemSampleTime=-1  VariantActivationTime=update diagram  Latency=0  AutoFrameSizeCalculation=off
      link override defval: Value=KINP_HMIACBtnCmd_flg_defval
      link override ovrdflg: Value=KINP_HMIACBtnCmd_flg_ovrdflg
      link override ovrdval: Value=KINP_HMIACBtnCmd_flg_ovrdval
  HMIACFrDefogBtnCmd : FVT_lib/inp/can_signal_template  SystemSampleTime=-1  VariantActivationTime=update diagram  Latency=0  AutoFrameSizeCalculation=off
      link override defval: Value=KINP_HMIACFrDefogBtnCmd_flg_defval
      link override ovrdflg: Value=KINP_HMIACFrDefogBtnCmd_flg_ovrdflg
      link override ovrdval: Value=KINP_HMIACFrDefogBtnCmd_flg_ovrdval
  HMIACRecycleBtnCmd : FVT_lib/inp/can_signal_template  SystemSampleTime=-1  VariantActivationTime=update diagram  Latency=0  AutoFrameSizeCalculation=off
      link override defval: Value=KINP_HMIACRecycleBtnCmd_flg_defval
      link override ovrdflg: Value=KINP_HMIACRecycleBtnCmd_flg_ovrdflg
      link override ovrdval: Value=KINP_HMIACRecycleBtnCmd_flg_ovrdval
  HMIACWindDirMCmd : FVT_lib/inp/can_signal_template  SystemSampleTime=-1  VariantActivationTime=update diagram  Latency=0  AutoFrameSizeCalculation=off
      link override defval: Value=KINP_HMIACWindDirMCmd_flg_defval
      link override ovrdflg: Value=KINP_HMIACWindDirMCmd_flg_ovrdflg
      link override ovrdval: Value=KINP_HMIACWindDirMCmd_flg_ovrdval
  HMIACWindDirPCmd : FVT_lib/inp/can_signal_template  SystemSampleTime=-1  VariantActivationTime=update diagram  Latency=0  AutoFrameSizeCalculation=off
      link override defval: Value=KINP_HMIACWindDirPCmd_flg_defval
      link override ovrdflg: Value=KINP_HMIACWindDirPCmd_flg_ovrdflg
      link override ovrdval: Value=KINP_HMIACWindDirPCmd_flg_ovrdval
  HMIAutoInterLightCmd : FVT_lib/inp/can_signal_template  SystemSampleTime=-1  VariantActivationTime=update diagram  Latency=0  AutoFrameSizeCalculation=off
      link override defval: Value=KINP_HMIAutoInterLightCmd_flg_defval
      link override ovrdflg: Value=KINP_HMIAutoInterLightCmd_flg_ovrdflg
      link override ovrdval: Value=KINP_HMIAutoInterLightCmd_flg_ovrdval
  HMIBCMPostDefogBtnCmd : FVT_lib/inp/can_signal_template  SystemSampleTime=-1  VariantActivationTime=update diagram  Latency=0  AutoFrameSizeCalculation=off
      link override defval: Value=KINP_HMIBCMPostDefogBtnCmd_flg_defval
      link override ovrdflg: Value=KINP_HMIBCMPostDefogBtnCmd_flg_ovrdflg
      link override ovrdval: Value=KINP_HMIBCMPostDefogBtnCmd_flg_ovrdval
  HMIZ1SetTMCmd : FVT_lib/inp/can_signal_template  SystemSampleTime=-1  VariantActivationTime=update diagram  Latency=0  AutoFrameSizeCalculation=off
      link override defval: Value=KINP_HMIZ1SetTMCmd_flg_defval
      link override ovrdflg: Value=KINP_HMIZ1SetTMCmd_flg_ovrdflg
      link override ovrdval: Value=KINP_HMIZ1SetTMCmd_flg_ovrdval
  HMIZ1SetTPCmd : FVT_lib/inp/can_signal_template  SystemSampleTime=-1  VariantActivationTime=update diagram  Latency=0  AutoFrameSizeCalculation=off
      link override defval: Value=KINP_HMIZ1SetTPCmd_flg_defval
      link override ovrdflg: Value=KINP_HMIZ1SetTPCmd_flg_ovrdflg
      link override ovrdval: Value=KINP_HMIZ1SetTPCmd_flg_ovrdval
  HMIZ2SetTMCmd : FVT_lib/inp/can_signal_template  SystemSampleTime=-1  VariantActivationTime=update diagram  Latency=0  AutoFrameSizeCalculation=off
      link override defval: Value=KINP_HMIZ2SetTMCmd_flg_defval
      link override ovrdflg: Value=KINP_HMIZ2SetTMCmd_flg_ovrdflg
      link override ovrdval: Value=KINP_HMIZ2SetTMCmd_flg_ovrdval
  HMIZ2SetTPCmd : FVT_lib/inp/can_signal_template  SystemSampleTime=-1  VariantActivationTime=update diagram  Latency=0  AutoFrameSizeCalculation=off
      link override defval: Value=KINP_HMIZ2SetTPCmd_flg_defval
      link override ovrdflg: Value=KINP_HMIZ2SetTPCmd_flg_ovrdflg
      link override ovrdval: Value=KINP_HMIZ2SetTPCmd_flg_ovrdval
  Terminator_{1..14} (14 alike) : Terminator
  True_VHAL_HMIACAirIntMCmd_flg : Constant  Value=TRUE  OutDataTypeStr=boolean
  True_VHAL_HMIACAirIntPCmd_flg : Constant  Value=TRUE  OutDataTypeStr=boolean
  True_VHAL_HMIACAutoBtnCmd_flg : Constant  Value=TRUE  OutDataTypeStr=boolean
  True_VHAL_HMIACBtnCmd_flg : Constant  Value=TRUE  OutDataTypeStr=boolean
  True_VHAL_HMIACFrDefogBtnCmd_flg : Constant  Value=TRUE  OutDataTypeStr=boolean
  True_VHAL_HMIACRecycleBtnCmd_flg : Constant  Value=TRUE  OutDataTypeStr=boolean
  True_VHAL_HMIACWindDirMCmd_flg : Constant  Value=TRUE  OutDataTypeStr=boolean
  True_VHAL_HMIACWindDirPCmd_flg : Constant  Value=TRUE  OutDataTypeStr=boolean
  True_VHAL_HMIAutoInterLightCmd_flg : Constant  Value=TRUE  OutDataTypeStr=boolean
  True_VHAL_HMIBCMPostDefogBtnCmd_flg : Constant  Value=TRUE  OutDataTypeStr=boolean
  True_VHAL_HMIZ1SetTMCmd_flg : Constant  Value=TRUE  OutDataTypeStr=boolean
  True_VHAL_HMIZ1SetTPCmd_flg : Constant  Value=TRUE  OutDataTypeStr=boolean
  True_VHAL_HMIZ2SetTMCmd_flg : Constant  Value=TRUE  OutDataTypeStr=boolean
  True_VHAL_HMIZ2SetTPCmd_flg : Constant  Value=TRUE  OutDataTypeStr=boolean
  slr1_{1..14} (14 alike) : BusSelector  OutputSignals=VINP_CANMsgValidHMI1_flg
  slr_VHAL_HMIACAirIntMCmd_flg : BusSelector  OutputSignals=VHAL_HMIACAirIntMCmd_flg
  slr_VHAL_HMIACAirIntPCmd_flg : BusSelector  OutputSignals=VHAL_HMIACAirIntPCmd_flg
  slr_VHAL_HMIACAutoBtnCmd_flg : BusSelector  OutputSignals=VHAL_HMIACAutoBtnCmd_flg
  slr_VHAL_HMIACBtnCmd_flg : BusSelector  OutputSignals=VHAL_HMIACBtnCmd_flg
  slr_VHAL_HMIACFrDefogBtnCmd_flg : BusSelector  OutputSignals=VHAL_HMIACFrDefogBtnCmd_flg
  slr_VHAL_HMIACRecycleBtnCmd_flg : BusSelector  OutputSignals=VHAL_HMIACRecycleBtnCmd_flg
  slr_VHAL_HMIACWindDirMCmd_flg : BusSelector  OutputSignals=VHAL_HMIACWindDirMCmd_flg
  slr_VHAL_HMIACWindDirPCmd_flg : BusSelector  OutputSignals=VHAL_HMIACWindDirPCmd_flg
  slr_VHAL_HMIAutoInterLightCmd_flg : BusSelector  OutputSignals=VHAL_HMIAutoInterLightCmd_flg
  slr_VHAL_HMIBCMPostDefogBtnCmd_flg : BusSelector  OutputSignals=VHAL_HMIBCMPostDefogBtnCmd_flg
  slr_VHAL_HMIZ1SetTMCmd_flg : BusSelector  OutputSignals=VHAL_HMIZ1SetTMCmd_flg
  slr_VHAL_HMIZ1SetTPCmd_flg : BusSelector  OutputSignals=VHAL_HMIZ1SetTPCmd_flg
  slr_VHAL_HMIZ2SetTMCmd_flg : BusSelector  OutputSignals=VHAL_HMIZ2SetTMCmd_flg
  slr_VHAL_HMIZ2SetTPCmd_flg : BusSelector  OutputSignals=VHAL_HMIZ2SetTPCmd_flg
  VINP_HMIACAirIntMCmd_flg : Outport
  VINP_HMIACAirIntPCmd_flg : Outport  Port=2
  VINP_HMIACAutoBtnCmd_flg : Outport  Port=3
  VINP_HMIACBtnCmd_flg : Outport  Port=4
  VINP_HMIACFrDefogBtnCmd_flg : Outport  Port=5
  VINP_HMIACRecycleBtnCmd_flg : Outport  Port=6
  VINP_HMIACWindDirMCmd_flg : Outport  Port=7
  VINP_HMIACWindDirPCmd_flg : Outport  Port=8
  VINP_HMIAutoInterLightCmd_flg : Outport  Port=9
  VINP_HMIBCMPostDefogBtnCmd_flg : Outport  Port=10
  VINP_HMIZ1SetTMCmd_flg : Outport  Port=11
  VINP_HMIZ1SetTPCmd_flg : Outport  Port=12
  VINP_HMIZ2SetTMCmd_flg : Outport  Port=13
  VINP_HMIZ2SetTPCmd_flg : Outport  Port=14
  wires:
  BHAL_outputs/1 -> [BHAL_outputs]
  inp_CanValid_bus/1 -> [inp_CanValid_bus]
  [BHAL_outputs] -> slr_VHAL_HMIACAirIntMCmd_flg/1
  slr_VHAL_HMIACAirIntMCmd_flg/1 -> HMIACAirIntMCmd/1  "<VHAL_HMIACAirIntMCmd_flg>"
  True_VHAL_HMIACAirIntMCmd_flg/1 -> HMIACAirIntMCmd/2
  [inp_CanValid_bus] -> slr1_1/1
  slr1_1/1 -> HMIACAirIntMCmd/3  "<VINP_CANMsgValidHMI1_flg>"
  HMIACAirIntMCmd/1 -> VINP_HMIACAirIntMCmd_flg/1  "VINP_HMIACAirIntMCmd_flg"
  HMIACAirIntMCmd/2 -> Terminator_1/1
  [BHAL_outputs] -> slr_VHAL_HMIACAirIntPCmd_flg/1
  slr_VHAL_HMIACAirIntPCmd_flg/1 -> HMIACAirIntPCmd/1  "<VHAL_HMIACAirIntPCmd_flg>"
  True_VHAL_HMIACAirIntPCmd_flg/1 -> HMIACAirIntPCmd/2
  [inp_CanValid_bus] -> slr1_2/1
  slr1_2/1 -> HMIACAirIntPCmd/3  "<VINP_CANMsgValidHMI1_flg>"
  HMIACAirIntPCmd/1 -> VINP_HMIACAirIntPCmd_flg/1  "VINP_HMIACAirIntPCmd_flg"
  HMIACAirIntPCmd/2 -> Terminator_2/1
  [BHAL_outputs] -> slr_VHAL_HMIACAutoBtnCmd_flg/1
  slr_VHAL_HMIACAutoBtnCmd_flg/1 -> HMIACAutoBtnCmd/1  "<VHAL_HMIACAutoBtnCmd_flg>"
  True_VHAL_HMIACAutoBtnCmd_flg/1 -> HMIACAutoBtnCmd/2
  [inp_CanValid_bus] -> slr1_3/1
  slr1_3/1 -> HMIACAutoBtnCmd/3  "<VINP_CANMsgValidHMI1_flg>"
  HMIACAutoBtnCmd/1 -> VINP_HMIACAutoBtnCmd_flg/1  "VINP_HMIACAutoBtnCmd_flg"
  HMIACAutoBtnCmd/2 -> Terminator_3/1
  [BHAL_outputs] -> slr_VHAL_HMIACBtnCmd_flg/1
  slr_VHAL_HMIACBtnCmd_flg/1 -> HMIACBtnCmd/1  "<VHAL_HMIACBtnCmd_flg>"
  True_VHAL_HMIACBtnCmd_flg/1 -> HMIACBtnCmd/2
  [inp_CanValid_bus] -> slr1_4/1
  slr1_4/1 -> HMIACBtnCmd/3  "<VINP_CANMsgValidHMI1_flg>"
  HMIACBtnCmd/1 -> VINP_HMIACBtnCmd_flg/1  "VINP_HMIACBtnCmd_flg"
  HMIACBtnCmd/2 -> Terminator_4/1
  [BHAL_outputs] -> slr_VHAL_HMIACFrDefogBtnCmd_flg/1
  slr_VHAL_HMIACFrDefogBtnCmd_flg/1 -> HMIACFrDefogBtnCmd/1  "<VHAL_HMIACFrDefogBtnCmd_flg>"
  True_VHAL_HMIACFrDefogBtnCmd_flg/1 -> HMIACFrDefogBtnCmd/2
  [inp_CanValid_bus] -> slr1_5/1
  slr1_5/1 -> HMIACFrDefogBtnCmd/3  "<VINP_CANMsgValidHMI1_flg>"
  HMIACFrDefogBtnCmd/1 -> VINP_HMIACFrDefogBtnCmd_flg/1  "VINP_HMIACFrDefogBtnCmd_flg"
  HMIACFrDefogBtnCmd/2 -> Terminator_5/1
  [BHAL_outputs] -> slr_VHAL_HMIACRecycleBtnCmd_flg/1
  slr_VHAL_HMIACRecycleBtnCmd_flg/1 -> HMIACRecycleBtnCmd/1  "<VHAL_HMIACRecycleBtnCmd_flg>"
  True_VHAL_HMIACRecycleBtnCmd_flg/1 -> HMIACRecycleBtnCmd/2
  [inp_CanValid_bus] -> slr1_6/1
  slr1_6/1 -> HMIACRecycleBtnCmd/3  "<VINP_CANMsgValidHMI1_flg>"
  HMIACRecycleBtnCmd/1 -> VINP_HMIACRecycleBtnCmd_flg/1  "VINP_HMIACRecycleBtnCmd_flg"
  HMIACRecycleBtnCmd/2 -> Terminator_6/1
  [BHAL_outputs] -> slr_VHAL_HMIACWindDirMCmd_flg/1
  slr_VHAL_HMIACWindDirMCmd_flg/1 -> HMIACWindDirMCmd/1  "<VHAL_HMIACWindDirMCmd_flg>"
  True_VHAL_HMIACWindDirMCmd_flg/1 -> HMIACWindDirMCmd/2
  [inp_CanValid_bus] -> slr1_7/1
  slr1_7/1 -> HMIACWindDirMCmd/3  "<VINP_CANMsgValidHMI1_flg>"
  HMIACWindDirMCmd/1 -> VINP_HMIACWindDirMCmd_flg/1  "VINP_HMIACWindDirMCmd_flg"
  HMIACWindDirMCmd/2 -> Terminator_7/1
  [BHAL_outputs] -> slr_VHAL_HMIACWindDirPCmd_flg/1
  slr_VHAL_HMIACWindDirPCmd_flg/1 -> HMIACWindDirPCmd/1  "<VHAL_HMIACWindDirPCmd_flg>"
  True_VHAL_HMIACWindDirPCmd_flg/1 -> HMIACWindDirPCmd/2
  [inp_CanValid_bus] -> slr1_8/1
  slr1_8/1 -> HMIACWindDirPCmd/3  "<VINP_CANMsgValidHMI1_flg>"
  HMIACWindDirPCmd/1 -> VINP_HMIACWindDirPCmd_flg/1  "VINP_HMIACWindDirPCmd_flg"
  HMIACWindDirPCmd/2 -> Terminator_8/1
  [BHAL_outputs] -> slr_VHAL_HMIAutoInterLightCmd_flg/1
  slr_VHAL_HMIAutoInterLightCmd_flg/1 -> HMIAutoInterLightCmd/1  "<VHAL_HMIAutoInterLightCmd_flg>"
  True_VHAL_HMIAutoInterLightCmd_flg/1 -> HMIAutoInterLightCmd/2
  [inp_CanValid_bus] -> slr1_9/1
  slr1_9/1 -> HMIAutoInterLightCmd/3  "<VINP_CANMsgValidHMI1_flg>"
  HMIAutoInterLightCmd/1 -> VINP_HMIAutoInterLightCmd_flg/1  "VINP_HMIAutoInterLightCmd_flg"
  HMIAutoInterLightCmd/2 -> Terminator_9/1
  [BHAL_outputs] -> slr_VHAL_HMIBCMPostDefogBtnCmd_flg/1
  slr_VHAL_HMIBCMPostDefogBtnCmd_flg/1 -> HMIBCMPostDefogBtnCmd/1  "<VHAL_HMIBCMPostDefogBtnCmd_flg>"
  True_VHAL_HMIBCMPostDefogBtnCmd_flg/1 -> HMIBCMPostDefogBtnCmd/2
  [inp_CanValid_bus] -> slr1_10/1
  slr1_10/1 -> HMIBCMPostDefogBtnCmd/3  "<VINP_CANMsgValidHMI1_flg>"
  HMIBCMPostDefogBtnCmd/1 -> VINP_HMIBCMPostDefogBtnCmd_flg/1  "VINP_HMIBCMPostDefogBtnCmd_flg"
  HMIBCMPostDefogBtnCmd/2 -> Terminator_10/1
  [BHAL_outputs] -> slr_VHAL_HMIZ1SetTMCmd_flg/1
  slr_VHAL_HMIZ1SetTMCmd_flg/1 -> HMIZ1SetTMCmd/1  "<VHAL_HMIZ1SetTMCmd_flg>"
  True_VHAL_HMIZ1SetTMCmd_flg/1 -> HMIZ1SetTMCmd/2
  [inp_CanValid_bus] -> slr1_11/1
  slr1_11/1 -> HMIZ1SetTMCmd/3  "<VINP_CANMsgValidHMI1_flg>"
  HMIZ1SetTMCmd/1 -> VINP_HMIZ1SetTMCmd_flg/1  "VINP_HMIZ1SetTMCmd_flg"
  HMIZ1SetTMCmd/2 -> Terminator_11/1
  [BHAL_outputs] -> slr_VHAL_HMIZ1SetTPCmd_flg/1
  slr_VHAL_HMIZ1SetTPCmd_flg/1 -> HMIZ1SetTPCmd/1  "<VHAL_HMIZ1SetTPCmd_flg>"
  True_VHAL_HMIZ1SetTPCmd_flg/1 -> HMIZ1SetTPCmd/2
  [inp_CanValid_bus] -> slr1_12/1
  slr1_12/1 -> HMIZ1SetTPCmd/3  "<VINP_CANMsgValidHMI1_flg>"
  HMIZ1SetTPCmd/1 -> VINP_HMIZ1SetTPCmd_flg/1  "VINP_HMIZ1SetTPCmd_flg"
  HMIZ1SetTPCmd/2 -> Terminator_12/1
  [BHAL_outputs] -> slr_VHAL_HMIZ2SetTMCmd_flg/1
  slr_VHAL_HMIZ2SetTMCmd_flg/1 -> HMIZ2SetTMCmd/1  "<VHAL_HMIZ2SetTMCmd_flg>"
  True_VHAL_HMIZ2SetTMCmd_flg/1 -> HMIZ2SetTMCmd/2
  [inp_CanValid_bus] -> slr1_13/1
  slr1_13/1 -> HMIZ2SetTMCmd/3  "<VINP_CANMsgValidHMI1_flg>"
  HMIZ2SetTMCmd/1 -> VINP_HMIZ2SetTMCmd_flg/1  "VINP_HMIZ2SetTMCmd_flg"
  HMIZ2SetTMCmd/2 -> Terminator_13/1
  [BHAL_outputs] -> slr_VHAL_HMIZ2SetTPCmd_flg/1
  slr_VHAL_HMIZ2SetTPCmd_flg/1 -> HMIZ2SetTPCmd/1  "<VHAL_HMIZ2SetTPCmd_flg>"
  True_VHAL_HMIZ2SetTPCmd_flg/1 -> HMIZ2SetTPCmd/2
  [inp_CanValid_bus] -> slr1_14/1
  slr1_14/1 -> HMIZ2SetTPCmd/3  "<VINP_CANMsgValidHMI1_flg>"
  HMIZ2SetTPCmd/1 -> VINP_HMIZ2SetTPCmd_flg/1  "VINP_HMIZ2SetTPCmd_flg"
  HMIZ2SetTPCmd/2 -> Terminator_14/1
